simulink model "backup"  (R2018b)
settings: Solver=VariableStepAuto  StartTime=0.0  StopTime=10.0  RelTol=1e-3
values from neighbouring files (symbols this model uses):
  b = 7.66E-5    (= 7.66e-05)    [drone.m]
  d = 5.63E-6    (= 5.63e-06)    [drone.m]
  g = 9.81    [drone.m]
  Ixx = 2.458E-4    (= 0.0002458)    [drone.m]
  Iyy = 4.090E-4    (= 0.000409)    [drone.m]
  Izz = 5.2256E-4    (= 0.00052256)    [drone.m]
  Jr = 5.225E-5    (= 5.225e-05)    [drone.m]
  l = 0.135    [drone.m]
  m = 0.494    [drone.m]
  Ts = 0.1    [drone.m]
undefined symbols (not defined in the file or in its folder): kd_phi, kd_psi, kd_theta, kd_z, ki_phi, ki_psi, ki_theta, ki_z, kp_phi, kp_psi, kp_theta, kp_z, ref
libraries: simulink x4
settings Model: Creator=Mauri  LastModifiedBy=Mauri

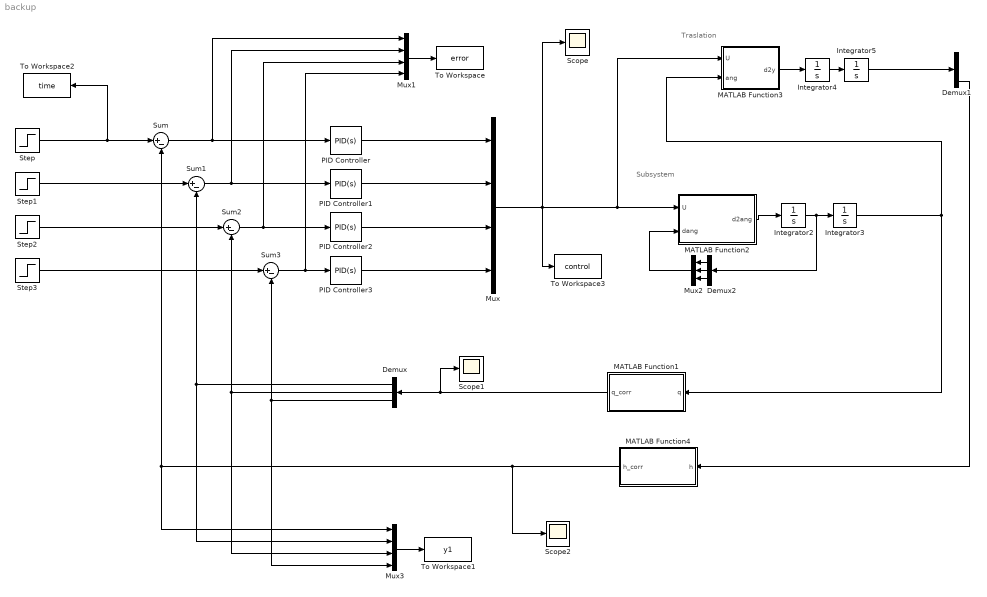
== system backup ==
  note: Subsystem
  note: Traslation
  Demux : Demux  Outputs=3
  Demux1 : Demux  Outputs=3
  Demux2 : Demux  Outputs=3
  Integrator{2..5} (4 alike) : Integrator  InitialCondition=0.01
  MATLAB Function1 : MATLAB Function  TreatAsAtomicUnit=on
  MATLAB Function2 : MATLAB Function  TreatAsAtomicUnit=on
  MATLAB Function3 : MATLAB Function  TreatAsAtomicUnit=on
  MATLAB Function4 : MATLAB Function  TreatAsAtomicUnit=on
  Mux : Mux
  Mux1 : Mux
  Mux2 : Mux  Inputs=3
  Mux3 : Mux
  PID Controller : simulink/Continuous/PID Controller  Controller=PID  Form=Parallel  TimeDomain=Continuous-time  SampleTime=-1  IntegratorMethod=Forward Euler  FilterMethod=Forward Euler  ControllerParametersSource=internal  P=kp_z  I=ki_z  D=kd_z  UseFilter=on  N=100  TunerSelectOption=Transfer Function Based (PID Tuner App)  InitialConditionSource=internal  InitialConditionForIntegrator=0  InitialConditionForFilter=0  DifferentiatorICPrevScaledInput=0  ExternalReset=none  TrackingMode=off  Kt=1  LimitOutput=off  UpperSaturationLimit=1000  LowerSaturationLimit=0  LinearizeAsGain=on  AntiWindupMode=none  Kb=1  POutMin=[]  POutMax=[]  IOutMin=[]  IOutMax=[]  DOutMin=[]  DOutMax=[]  NOutMin=[]  NOutMax=[]  SumOutMin=[]  SumOutMax=[]  SaturationOutMin=[]  SaturationOutMax=[]  PParamMin=[]  PParamMax=[]  IParamMin=[]  IParamMax=[]  DParamMin=[]  DParamMax=[]  NParamMin=[]  NParamMax=[]  KbParamMin=[]  KbParamMax=[]  KtParamMin=[]  KtParamMax=[]  KbOutMin=[]  KbOutMax=[]  KtOutMin=[]  KtOutMax=[]  IntegratorOutMin=[]  IntegratorOutMax=[]  FilterOutMin=[]  FilterOutMax=[]  SumI1OutMin=[]  SumI1OutMax=[]  SumI2OutMin=[]  SumI2OutMax=[]  SumI3OutMin=[]  SumI3OutMax=[]  SumI4OutMin=[]  SumI4OutMax=[]  SumDOutMin=[]  SumDOutMax=[]  DifferentiatorOutMin=[]  DifferentiatorOutMax=[]  FilterDiffOutCoefMin=[]  FilterDiffOutCoefMax=[]  ReciprocalOutMin=[]  ReciprocalOutMax=[]  SumDenOutMin=[]  SumDenOutMax=[]  SumNumOutMin=[]  SumNumOutMax=[]  DivideOutMin=[]  DivideOutMax=[]  IntegratorContinuousStateAttributes=''  IntegratorStateMustResolveToSignalObject=off  IntegratorRTWStateStorageClass=Auto  FilterContinuousStateAttributes=''  FilterStateMustResolveToSignalObject=off  FilterRTWStateStorageClass=Auto  ParallelPVariant=InternalParameters  IdealPVariant=Disabled  IVariant=InternalParameters  DVariant=InternalParameters  IntegratorVariant=Continuous  SatVariant=Disabled  AWVariant=Passthrough  PCopyVariant=Disabled  TRVariant=Disabled  FdbkBlocksVariant=Forward  IdealPFdbkVariant=Disabled  SatFdbkVariant=Disabled  DerivativeFilterVariant=ContFilter  NVariant=InternalParameters  NCopyVariant=Disabled  FilterICVariant=InternalICsFilter  IntegratorICVariant=InternalICs  ExternalResetVariant=Disabled  TRSumVariant=Passthrough  SumFdbkVariant=Disabled  SumVariant=Sum_PID
  PID Controller1 : simulink/Continuous/PID Controller  Controller=PID  Form=Parallel  TimeDomain=Continuous-time  SampleTime=-1  IntegratorMethod=Forward Euler  FilterMethod=Forward Euler  ControllerParametersSource=internal  P=kp_phi  I=ki_phi  D=kd_phi  UseFilter=on  N=100  TunerSelectOption=Transfer Function Based (PID Tuner App)  InitialConditionSource=internal  InitialConditionForIntegrator=0  InitialConditionForFilter=0  DifferentiatorICPrevScaledInput=0  ExternalReset=none  TrackingMode=off  Kt=1  LimitOutput=off  UpperSaturationLimit=1000  LowerSaturationLimit=-1000  LinearizeAsGain=on  AntiWindupMode=none  Kb=1  POutMin=[]  POutMax=[]  IOutMin=[]  IOutMax=[]  DOutMin=[]  DOutMax=[]  NOutMin=[]  NOutMax=[]  SumOutMin=[]  SumOutMax=[]  SaturationOutMin=[]  SaturationOutMax=[]  PParamMin=[]  PParamMax=[]  IParamMin=[]  IParamMax=[]  DParamMin=[]  DParamMax=[]  NParamMin=[]  NParamMax=[]  KbParamMin=[]  KbParamMax=[]  KtParamMin=[]  KtParamMax=[]  KbOutMin=[]  KbOutMax=[]  KtOutMin=[]  KtOutMax=[]  IntegratorOutMin=[]  IntegratorOutMax=[]  FilterOutMin=[]  FilterOutMax=[]  SumI1OutMin=[]  SumI1OutMax=[]  SumI2OutMin=[]  SumI2OutMax=[]  SumI3OutMin=[]  SumI3OutMax=[]  SumI4OutMin=[]  SumI4OutMax=[]  SumDOutMin=[]  SumDOutMax=[]  DifferentiatorOutMin=[]  DifferentiatorOutMax=[]  FilterDiffOutCoefMin=[]  FilterDiffOutCoefMax=[]  ReciprocalOutMin=[]  ReciprocalOutMax=[]  SumDenOutMin=[]  SumDenOutMax=[]  SumNumOutMin=[]  SumNumOutMax=[]  DivideOutMin=[]  DivideOutMax=[]  IntegratorContinuousStateAttributes=''  IntegratorStateMustResolveToSignalObject=off  IntegratorRTWStateStorageClass=Auto  FilterContinuousStateAttributes=''  FilterStateMustResolveToSignalObject=off  FilterRTWStateStorageClass=Auto  ParallelPVariant=InternalParameters  IdealPVariant=Disabled  IVariant=InternalParameters  DVariant=InternalParameters  IntegratorVariant=Continuous  SatVariant=Disabled  AWVariant=Passthrough  PCopyVariant=Disabled  TRVariant=Disabled  FdbkBlocksVariant=Forward  IdealPFdbkVariant=Disabled  SatFdbkVariant=Disabled  DerivativeFilterVariant=ContFilter  NVariant=InternalParameters  NCopyVariant=Disabled  FilterICVariant=InternalICsFilter  IntegratorICVariant=InternalICs  ExternalResetVariant=Disabled  TRSumVariant=Passthrough  SumFdbkVariant=Disabled  SumVariant=Sum_PID
  PID Controller2 : simulink/Continuous/PID Controller  Controller=PID  Form=Parallel  TimeDomain=Continuous-time  SampleTime=-1  IntegratorMethod=Forward Euler  FilterMethod=Forward Euler  ControllerParametersSource=internal  P=kp_theta  I=ki_theta  D=kd_theta  UseFilter=on  N=100  TunerSelectOption=Transfer Function Based (PID Tuner App)  InitialConditionSource=internal  InitialConditionForIntegrator=0  InitialConditionForFilter=0  DifferentiatorICPrevScaledInput=0  ExternalReset=none  TrackingMode=off  Kt=1  LimitOutput=off  UpperSaturationLimit=1000  LowerSaturationLimit=-1000  LinearizeAsGain=on  AntiWindupMode=none  Kb=1  POutMin=[]  POutMax=[]  IOutMin=[]  IOutMax=[]  DOutMin=[]  DOutMax=[]  NOutMin=[]  NOutMax=[]  SumOutMin=[]  SumOutMax=[]  SaturationOutMin=[]  SaturationOutMax=[]  PParamMin=[]  PParamMax=[]  IParamMin=[]  IParamMax=[]  DParamMin=[]  DParamMax=[]  NParamMin=[]  NParamMax=[]  KbParamMin=[]  KbParamMax=[]  KtParamMin=[]  KtParamMax=[]  KbOutMin=[]  KbOutMax=[]  KtOutMin=[]  KtOutMax=[]  IntegratorOutMin=[]  IntegratorOutMax=[]  FilterOutMin=[]  FilterOutMax=[]  SumI1OutMin=[]  SumI1OutMax=[]  SumI2OutMin=[]  SumI2OutMax=[]  SumI3OutMin=[]  SumI3OutMax=[]  SumI4OutMin=[]  SumI4OutMax=[]  SumDOutMin=[]  SumDOutMax=[]  DifferentiatorOutMin=[]  DifferentiatorOutMax=[]  FilterDiffOutCoefMin=[]  FilterDiffOutCoefMax=[]  ReciprocalOutMin=[]  ReciprocalOutMax=[]  SumDenOutMin=[]  SumDenOutMax=[]  SumNumOutMin=[]  SumNumOutMax=[]  DivideOutMin=[]  DivideOutMax=[]  IntegratorContinuousStateAttributes=''  IntegratorStateMustResolveToSignalObject=off  IntegratorRTWStateStorageClass=Auto  FilterContinuousStateAttributes=''  FilterStateMustResolveToSignalObject=off  FilterRTWStateStorageClass=Auto  ParallelPVariant=InternalParameters  IdealPVariant=Disabled  IVariant=InternalParameters  DVariant=InternalParameters  IntegratorVariant=Continuous  SatVariant=Disabled  AWVariant=Passthrough  PCopyVariant=Disabled  TRVariant=Disabled  FdbkBlocksVariant=Forward  IdealPFdbkVariant=Disabled  SatFdbkVariant=Disabled  DerivativeFilterVariant=ContFilter  NVariant=InternalParameters  NCopyVariant=Disabled  FilterICVariant=InternalICsFilter  IntegratorICVariant=InternalICs  ExternalResetVariant=Disabled  TRSumVariant=Passthrough  SumFdbkVariant=Disabled  SumVariant=Sum_PID
  PID Controller3 : simulink/Continuous/PID Controller  Controller=PID  Form=Parallel  TimeDomain=Continuous-time  SampleTime=-1  IntegratorMethod=Forward Euler  FilterMethod=Forward Euler  ControllerParametersSource=internal  P=kp_psi  I=ki_psi  D=kd_psi  UseFilter=on  N=100  TunerSelectOption=Transfer Function Based (PID Tuner App)  InitialConditionSource=internal  InitialConditionForIntegrator=0  InitialConditionForFilter=0  DifferentiatorICPrevScaledInput=0  ExternalReset=none  TrackingMode=off  Kt=1  LimitOutput=off  UpperSaturationLimit=1000  LowerSaturationLimit=-1000  LinearizeAsGain=on  AntiWindupMode=none  Kb=1  POutMin=[]  POutMax=[]  IOutMin=[]  IOutMax=[]  DOutMin=[]  DOutMax=[]  NOutMin=[]  NOutMax=[]  SumOutMin=[]  SumOutMax=[]  SaturationOutMin=[]  SaturationOutMax=[]  PParamMin=[]  PParamMax=[]  IParamMin=[]  IParamMax=[]  DParamMin=[]  DParamMax=[]  NParamMin=[]  NParamMax=[]  KbParamMin=[]  KbParamMax=[]  KtParamMin=[]  KtParamMax=[]  KbOutMin=[]  KbOutMax=[]  KtOutMin=[]  KtOutMax=[]  IntegratorOutMin=[]  IntegratorOutMax=[]  FilterOutMin=[]  FilterOutMax=[]  SumI1OutMin=[]  SumI1OutMax=[]  SumI2OutMin=[]  SumI2OutMax=[]  SumI3OutMin=[]  SumI3OutMax=[]  SumI4OutMin=[]  SumI4OutMax=[]  SumDOutMin=[]  SumDOutMax=[]  DifferentiatorOutMin=[]  DifferentiatorOutMax=[]  FilterDiffOutCoefMin=[]  FilterDiffOutCoefMax=[]  ReciprocalOutMin=[]  ReciprocalOutMax=[]  SumDenOutMin=[]  SumDenOutMax=[]  SumNumOutMin=[]  SumNumOutMax=[]  DivideOutMin=[]  DivideOutMax=[]  IntegratorContinuousStateAttributes=''  IntegratorStateMustResolveToSignalObject=off  IntegratorRTWStateStorageClass=Auto  FilterContinuousStateAttributes=''  FilterStateMustResolveToSignalObject=off  FilterRTWStateStorageClass=Auto  ParallelPVariant=InternalParameters  IdealPVariant=Disabled  IVariant=InternalParameters  DVariant=InternalParameters  IntegratorVariant=Continuous  SatVariant=Disabled  AWVariant=Passthrough  PCopyVariant=Disabled  TRVariant=Disabled  FdbkBlocksVariant=Forward  IdealPFdbkVariant=Disabled  SatFdbkVariant=Disabled  DerivativeFilterVariant=ContFilter  NVariant=InternalParameters  NCopyVariant=Disabled  FilterICVariant=InternalICsFilter  IntegratorICVariant=InternalICs  ExternalResetVariant=Disabled  TRSumVariant=Passthrough  SumFdbkVariant=Disabled  SumVariant=Sum_PID
  Scope : Scope
  Scope1 : Scope
  Scope2 : Scope
  Step : Step  Time=step(1)  After=ref(1)  SampleTime=0
  Step1 : Step  Time=step(2)  After=ref(2)  SampleTime=0
  Step2 : Step  Time=step(3)  After=ref(3)  SampleTime=0
  Step3 : Step  Time=step(4)  After=ref(4)  SampleTime=0
  Sum{,1..3} (4 alike) : Sum  Inputs=|+-
  To Workspace : ToWorkspace  VariableName=error  SampleTime=Ts
  To Workspace1 : ToWorkspace  VariableName=y1  SampleTime=Ts
  To Workspace2 : ToWorkspace  VariableName=time  SaveFormat=Timeseries  SampleTime=Ts
  To Workspace3 : ToWorkspace  VariableName=control  SampleTime=Ts
  wires:
  Step3/1 -> Sum3/1
  PID Controller/1 -> Mux/1
  PID Controller2/1 -> Mux/3
  Integrator5/1 -> Demux1/1
  MATLAB Function3/1(d2y) -> Integrator4/1
  Integrator4/1 -> Integrator5/1
  MATLAB Function1/1(q_corr) -> Demux/1, Scope1/1
  Demux/1 -> Mux3/2, Sum1/2
  Integrator3/1 -> MATLAB Function1/1(q), MATLAB Function3/2(ang)
  Mux3/1 -> To Workspace1/1
  Demux2/1 -> Mux2/1
  MATLAB Function2/1(d2ang) -> Integrator2/1
  Sum3/1 -> Mux1/4, PID Controller3/1
  Sum/1 -> Mux1/1, PID Controller/1
  Mux2/1 -> MATLAB Function2/2(dang)
  Integrator2/1 -> Demux2/1, Integrator3/1
  Demux/2 -> Sum2/2, Mux3/3
  Mux1/1 -> To Workspace/1
  Mux/1 -> Scope/1, MATLAB Function3/1(U), MATLAB Function2/1(U), To Workspace3/1
  Sum1/1 -> Mux1/2, PID Controller1/1
  MATLAB Function4/1(h_corr) -> Scope2/1, Sum/2, Mux3/1
  PID Controller3/1 -> Mux/4
  Step1/1 -> Sum1/1
  Demux2/3 -> Mux2/3
  Demux/3 -> Sum3/2, Mux3/4
  Demux1/3 -> MATLAB Function4/1(h)
  Sum2/1 -> Mux1/3, PID Controller2/1
  Step/1 -> To Workspace2/1, Sum/1
  PID Controller1/1 -> Mux/2
  Step2/1 -> Sum2/1
  Demux2/2 -> Mux2/2

== matlab function backup/MATLAB Function1 ==
  data: q input size=3,1; q_corr output size=3,1
function q_corr = limit_angles(q)
% Euler angles between the range of [-2*pi 2*pi]
q_corr = q;
for i=1:3
   if(abs(q(i)) >= 2*pi)
       q_corr(i) = mod(q(i),2*pi);
   else
       q_corr(i) = q(i);
   end
end
% Limit the angles on the range of [-pi pi]
for i=1:3
   if(q_corr(i) >= pi)
       q_corr(i) = q_corr(i)-2*pi;
   else
     if (q_corr(i) <= -pi)
       q_corr(i) = q_corr(i)+2*pi;
     end
   end  
end

== matlab function backup/MATLAB Function4 ==
  data: h input size=1,1; h_corr output size=1,1
function h_corr = limit_high(h)
% Euler angles between the range of [-2*pi 2*pi]
if(h < 0)
       h_corr = 0;
else
      h_corr = h;
end

== matlab function backup/MATLAB Function2 ==
  data: U input double size=4,1; d2ang output double size=3,1; dang input size=3,1; l parameter; Ixx parameter; Iyy parameter; Izz parameter; Jr parameter; b parameter; d parameter
function d2ang = rotation(U,dang, l, Ixx, Iyy, Izz, Jr, b, d)
% function that determines the translational movement of the drone.
% x: Rotor speed vector (x1,x2,x3,x4)
% ang: Roll(phi) Pitch(theta) Yaw(psi)
% z: aceleration of the coordenates axis.

l=0.22;  % m
Ixx=8.5532E-3;  
Iyy=8.5532E-3;  
Izz=1.476E-2;

Jr=5.225E-5;
b=7.66E-5;  % Thrust coefficient
d=5.63E-6;  % Drag coefficient

dphi=dang(1);
dtheta=dang(2);
dpsi=dang(3);
% Calculate ohm.
% ohm2=([b*[1 1 1 1];l*b*[0 -1 0 1];l*b*[-1 0 1 0];d*[-1 1 -1 1]])\U;
ohm2=([b*[1 1 1 1];l*b*[0 1 0 -1];l*b*[-1 0 1 0];d*[-1 1 -1 1]])\U;

% ohm2=M*U;
for i=1:4
    if (ohm2(i)<= 0)
        ohm2(i)=0;
    end
end    
ohm=sqrt(ohm2);
%ohmr=-ohm(1)+ohm(2)-ohm(3)+ohm(4);
ohmr=ohm(1)-ohm(2)+ohm(3)-ohm(4);
% ohm=-sqrt(abs(x(1)))+sqrt(abs(x(2)))-sqrt(abs(x(3)))+sqrt(abs(x(4)))
% ohm=-x(1)+x(2)-x(3)+x(4);
% d2ang=[1/Ixx*(dtheta*dpsi*(-Izz+Iyy)-dtheta*ohmr*Jr+U(2));...
%     1/Iyy*(dphi*dpsi*(-Ixx+Izz)+dphi*ohmr*Jr+U(3));...
%     1/Izz*(dphi*dtheta*(Ixx-Iyy)+U(4))];
 d2ang=[1/Ixx*(dtheta*dpsi*(-Izz+Iyy)+dtheta*ohmr*Jr+U(2));...
     1/Iyy*(dphi*dpsi*(-Ixx+Izz)-dphi*ohmr*Jr+U(3));...
     1/Izz*(dphi*dtheta*(-Iyy+Ixx)+ohmr*Jr+U(4))];

== matlab function backup/MATLAB Function3 ==
  data: U input size=4,1; d2y output size=3,1; ang input size=3,1; m parameter; g parameter
function d2y = fcn(U,ang, m, g)
% m=0.964;     % Kg
% g=9.81;      % Gravety m/s*2

phi=ang(1);
theta=ang(2);
psi=ang(3);
%d2y=[U(1)/m*(-sin(theta)*cos(phi));... % Datos paper
%      U(1)/m*(sin(phi));...
%      -g+cos(theta)*cos(phi)*U(1)/m];
  d2y=[U(1)/m*(sin(psi)*sin(phi)+cos(psi)*sin(theta)*cos(phi));... % Datos tesis
     U(1)/m*(-cos(psi)*sin(phi)+sin(psi)*sin(theta)*cos(phi));...
     -g+cos(theta)*cos(phi)*U(1)/m];
